simulink model "terrainfollow_sim_OLD"  (R2018a)
settings: Solver=VariableStepAuto  StartTime=0.0  StopTime=60  RelTol=1e-3
values from neighbouring files (symbols this model uses):
  A = [0 0 0.00013165266625 3.15369085605e-06 -1.52707114267e-20 299.999999993 0 -32.1699999992 -6.02299064272e-14 0 0 0 ... (25 elements, 5x5)]    [redu_ss_terrainfollow.mat]    (also in reducefun_terrainfollow.m = A_longitude_lo(1:5,1:5))
  B = [0  0; 0  0; 0.00154396044469  -0.00453382204302; -9.49308816068e-07  -0.00111635553349; 0  -0.0570163434913]    [redu_ss_terrainfollow.mat]    (also in reducefun_terrainfollow.m = A_longitude_lo(1:5,[6 7]))
  C = [1 0 0 0 0 0 1 0 0 0 0 0 ... (25 elements, 5x5)]    [redu_ss_terrainfollow.mat]    (also in reducefun_terrainfollow.m = eye(5))
  D = [0  0; 0  0; 0  0; 0  0; 0  0]    [redu_ss_terrainfollow.mat]    (also in reducefun_terrainfollow.m = zeros(5,2))
  ele_lowlim = -25    - de0    [terrainfollow_run.m]    (also in terrainfollow_sim_bigcanyon.m)
  ele_uplim = 25     - de0    [terrainfollow_run.m]    (also in terrainfollow_sim_bigcanyon.m)
  gclear = 40    [terrainfollow_run.m]    (also in terrainfollow_sim_bigcanyon.m)
  h0 = 1500    [terrainfollow_run.m]    (also in terrainfollow_sim_bigcanyon.m)
  K_i = K_f(:,2:5)    [terrainfollow_run.m]    (also in terrainfollow_sim_bigcanyon.m)
  K_o = K_f(:,1)    [terrainfollow_run.m]    (also in terrainfollow_sim_bigcanyon.m)
  th_lowlim = 1000   - th0    [terrainfollow_run.m]    (also in terrainfollow_sim_bigcanyon.m)
  th_uplim = 19000  - th0    [terrainfollow_run.m]    (also in terrainfollow_sim_bigcanyon.m)
  v0 = ft2m*trim_state_lo(7)    [terrainfollow_run.m]    (also in terrainfollow_sim_bigcanyon.m)
undefined symbols (not defined in the file or in its folder): trim_control_lo, trim_thrust_lo
settings Model: Creator=Lukas  LastModifiedBy=Lukas
settings CodeAppCC: StateflowObjectComments=on

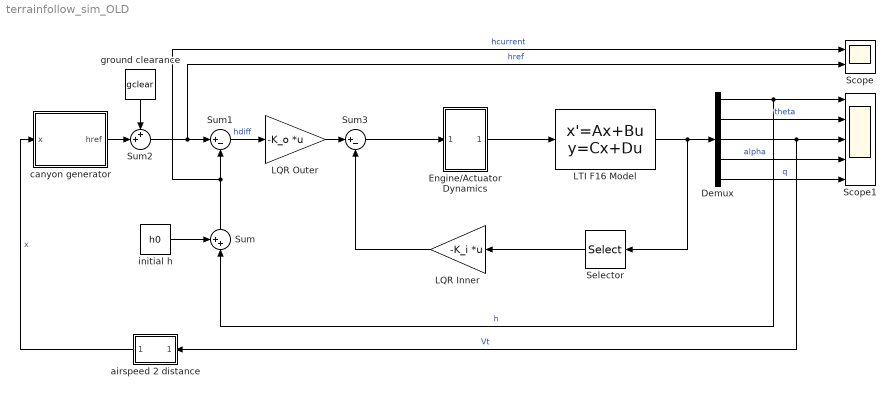
== system terrainfollow_sim_OLD ==
  Demux : Demux  Outputs=5
  Engine/Actuator Dynamics : Subsystem
  LQR Inner : Gain  Gain=-K_i  Multiplication=Matrix(K*u)  SaturateOnIntegerOverflow=on  OutDataTypeStr=Inherit: Same as input  ParamDataTypeStr=Inherit: Same as input
  LQR Outer : Gain  Gain=-K_o  Multiplication=Matrix(K*u)  SaturateOnIntegerOverflow=on  OutDataTypeStr=Inherit: Same as input  ParamDataTypeStr=Inherit: Same as input
  "LTI F16 Model " : StateSpace  A=A  B=B  C=C  D=D  InitialCondition=0
      mask Display: image('f16thumb.jpg');
  Scope : Scope  NumInputPorts=2
  Scope1 : Scope  NumInputPorts=5
  Selector : Selector  InputPortWidth=5  IndexOptions=Index vector (dialog)  Indices=[2 3 4 5]  OutputSizes=1
  Sum : Sum  Inputs=++|
  Sum1 : Sum  Inputs=|+-
  Sum2 : Sum  Inputs=++|
  Sum3 : Sum  Inputs=|+-
  airspeed 2 distance : Subsystem
  canyon generator : Subsystem
      mask Display: image(imread('canyon.jpg'))
  ground clearance : Constant  Value=gclear
  initial h : Constant  Value=h0
  wires:
  ground clearance/1 -> Sum2/1
  Sum1/1 -> LQR Outer/1  "hdiff"
  canyon generator/1(href) -> Sum2/2
  initial h/1 -> Sum/1
  airspeed 2 distance/1(Out1) -> canyon generator/1(x)  "x"
  Sum2/1 -> Scope/2, Sum1/1  "href"
  Demux/1 -> Scope1/1, Sum/2  "h"
  Demux/4 -> Scope1/4  "alpha"
  Demux/2 -> Scope1/2  "theta"
  Demux/3 -> airspeed 2 distance/1(In1), Scope1/3  "Vt"
  Demux/5 -> Scope1/5  "q"
  LQR Outer/1 -> Sum3/1
  LQR Inner/1 -> Sum3/2
  Sum3/1 -> Engine/Actuator Dynamics/1(In1)
  Engine/Actuator Dynamics/1(Out1) -> "LTI F16 Model "/1
  "LTI F16 Model "/1 -> Selector/1, Demux/1
  Selector/1 -> LQR Inner/1
  Sum/1 -> Scope/1, Sum1/2  "hcurrent"

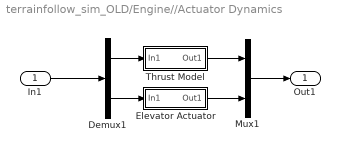
== system terrainfollow_sim_OLD/Engine//Actuator Dynamics ==
  In1 : Inport
  Demux1 : Demux  Outputs=2
  Elevator Actuator : Subsystem  AncestorBlock=F16_Actuator_Library/Elevator Actuator
  Mux1 : Mux  Inputs=2
  Thrust Model : Subsystem  AncestorBlock=F16_Actuator_Library/Thrust Model
  Out1 : Outport
  wires:
  In1/1 -> Demux1/1
  Demux1/2 -> Elevator Actuator/1(In1)
  Demux1/1 -> Thrust Model/1(In1)
  Thrust Model/1(Out1) -> Mux1/1
  Elevator Actuator/1(Out1) -> Mux1/2
  Mux1/1 -> Out1/1

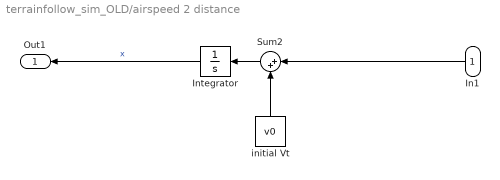
== system terrainfollow_sim_OLD/airspeed 2 distance ==
  In1 : Inport
  Integrator : Integrator
  Sum2 : Sum  Inputs=|++
  initial Vt : Constant  Value=v0
  Out1 : Outport
  wires:
  initial Vt/1 -> Sum2/2
  In1/1 -> Sum2/1
  Integrator/1 -> Out1/1  "x"
  Sum2/1 -> Integrator/1

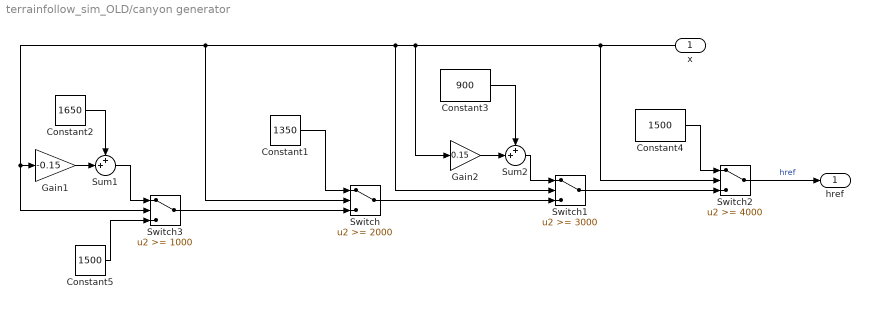
== system terrainfollow_sim_OLD/canyon generator ==
  x : Inport
  Constant1 : Constant  Value=1350
  Constant2 : Constant  Value=1650
  Constant3 : Constant  Value=900
  Constant4 : Constant  Value=1500
  Constant5 : Constant  Value=1500
  Gain1 : Gain  Gain=-0.15
  Gain2 : Gain  Gain=0.15
  Sum1 : Sum  Inputs=++|
  Sum2 : Sum  Inputs=++|
  Switch : Switch  Threshold=2000  ZeroCross=off
  Switch1 : Switch  Threshold=3000  ZeroCross=off
  Switch2 : Switch  Threshold=4000  ZeroCross=off
  Switch3 : Switch  Threshold=1000  ZeroCross=off
  href : Outport
  wires:
  Constant1/1 -> Switch/1
  x/1 -> Switch2/2, Gain2/1, Switch1/2, Switch/2, Gain1/1, Switch3/2
  Switch/1 -> Switch1/3
  Gain2/1 -> Sum2/2
  Constant3/1 -> Sum2/1
  Sum2/1 -> Switch1/1
  Switch1/1 -> Switch2/3
  Constant4/1 -> Switch2/1
  Switch2/1 -> href/1  "href"
  Switch3/1 -> Switch/3
  Constant5/1 -> Switch3/3
  Sum1/1 -> Switch3/1
  Gain1/1 -> Sum1/2
  Constant2/1 -> Sum1/1

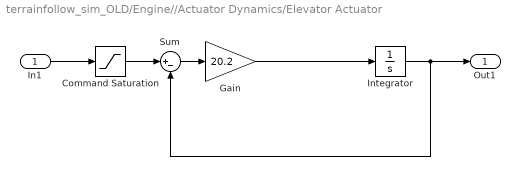
== system terrainfollow_sim_OLD/Engine//Actuator Dynamics/Elevator Actuator ==
  In1 : Inport
  " Command Saturation " : Saturate  UpperLimit=ele_uplim  LowerLimit=ele_lowlim
  Gain : Gain  Gain=20.2  SaturateOnIntegerOverflow=on  OutDataTypeStr=Inherit: Same as input  ParamDataTypeStr=Inherit: Same as input
  "Integrator " : Integrator  InitialCondition=trim_control_lo(1)  UpperSaturationLimit=25  LowerSaturationLimit=-25
  Sum : Sum  Inputs=|+-  SaturateOnIntegerOverflow=on  InputSameDT=on  OutDataTypeStr=Inherit: Same as first input
  Out1 : Outport
  wires:
  "Integrator "/1 -> Sum/2, Out1/1
  Gain/1 -> "Integrator "/1
  Sum/1 -> Gain/1
  In1/1 -> " Command Saturation "/1
  " Command Saturation "/1 -> Sum/1

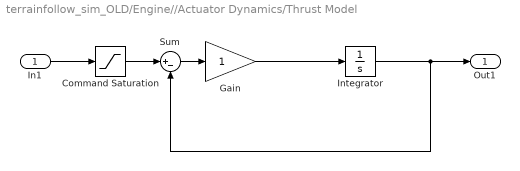
== system terrainfollow_sim_OLD/Engine//Actuator Dynamics/Thrust Model ==
  In1 : Inport
  " Command Saturation " : Saturate  UpperLimit=th_uplim  LowerLimit=th_lowlim
  Gain : Gain  SaturateOnIntegerOverflow=on  OutDataTypeStr=Inherit: Same as input  ParamDataTypeStr=Inherit: Same as input
  "Integrator " : Integrator  InitialCondition=trim_thrust_lo  UpperSaturationLimit=30  LowerSaturationLimit=-30
  Sum : Sum  Inputs=|+-  SaturateOnIntegerOverflow=on  InputSameDT=on  OutDataTypeStr=Inherit: Same as first input
  Out1 : Outport
  wires:
  "Integrator "/1 -> Sum/2, Out1/1
  Gain/1 -> "Integrator "/1
  Sum/1 -> Gain/1
  In1/1 -> " Command Saturation "/1
  " Command Saturation "/1 -> Sum/1
